simulink model "ARI_26_2_Integrator_Nonlinear2_JF"  (Simulink 7.8)
settings: Solver=ode45  StartTime=0.0  StopTime=5  MaxStep=.05  RelTol=1e-9
settings Model: Creator=Jindra Fuka  LastModifiedBy=Michael
settings OptimizationCC: InitFltsAndDblsToZero=on
settings DebuggingCC: FcnCallInpInsideContextMsg=Use local settings  StrictBusMsg=Warning

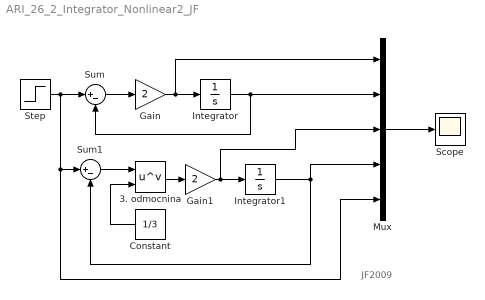
== system ARI_26_2_Integrator_Nonlinear2_JF ==
  note: JF2009
  3. odmocnina : Math  Operator=pow  SaturateOnIntegerOverflow=on
  Constant : Constant  Value=1/3
  Gain : Gain  Gain=2
  Gain1 : Gain  Gain=2
  Integrator : Integrator
  Integrator1 : Integrator  AbsoluteTolerance=1e-9
  Mux : Mux  Inputs=5
  Scope : Scope
      settings: TimeRange=5  YMin=2.77556e-017  YMax=1  MaxDataPoints=5000000
  Step : Step  SampleTime=0
  Sum : Sum  Inputs=|+-
  Sum1 : Sum  Inputs=|+-
  wires:
  Step/1 -> Sum/1, Sum1/1, Mux/5
  Sum/1 -> Gain/1
  Gain/1 -> Integrator/1, Mux/1
  Integrator/1 -> Mux/2, Sum/2
  Mux/1 -> Scope/1
  Gain1/1 -> Integrator1/1, Mux/3
  Integrator1/1 -> Mux/4, Sum1/2
  Sum1/1 -> 3. odmocnina/1
  3. odmocnina/1 -> Gain1/1
  Constant/1 -> 3. odmocnina/2
